simulink model "InverseDynamicsController"  (R2020b)
settings: Solver=FixedStepAuto  StartTime=0.0  StopTime=42  RelTol=1e-3
settings Model: Creator=Riley  LastModifiedBy=Riley

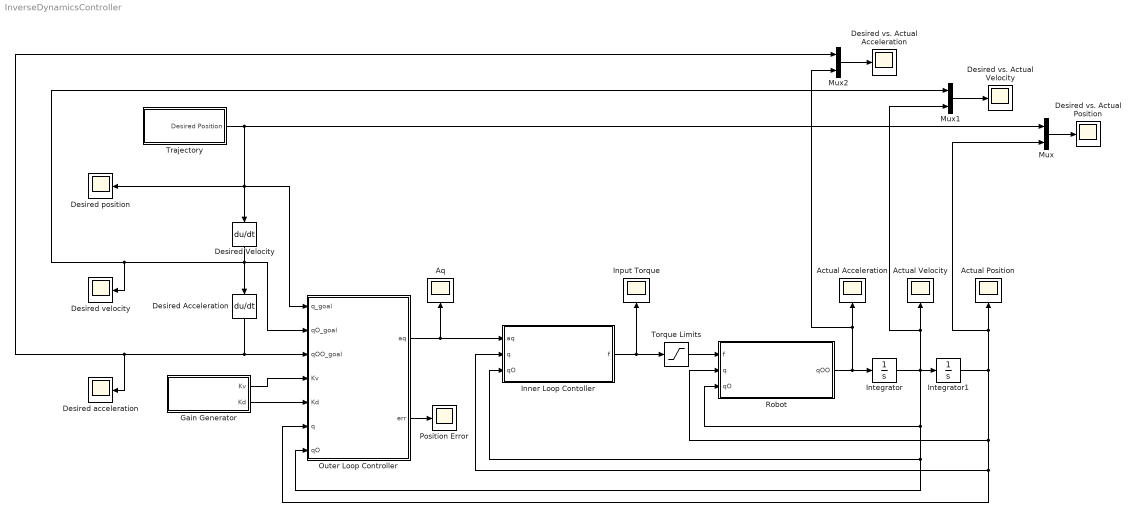
== system InverseDynamicsController ==
  Actual Acceleration : Scope
  Actual Position : Scope
  Actual Velocity : Scope
  Aq : Scope
  Desired Acceleration : Derivative
  Desired Velocity : Derivative
  Desired acceleration : Scope
  Desired position : Scope
  Desired velocity : Scope
  Desired vs. Actual Acceleration : Scope
  Desired vs. Actual Position : Scope
  Desired vs. Actual Velocity : Scope
  Gain Generator : Subsystem
  Inner Loop Contoller : MATLAB Function  TreatAsAtomicUnit=on
  Input Torque : Scope
  Integrator : Integrator  InitialCondition=[0,0,0]
  Integrator1 : Integrator  InitialCondition=[0,0,0]
  Mux : Mux  Inputs=2
  Mux1 : Mux  Inputs=2
  Mux2 : Mux  Inputs=2
  Outer Loop Controller : MATLAB Function  TreatAsAtomicUnit=on
  Position Error : Scope
  Robot : MATLAB Function  TreatAsAtomicUnit=on
  Torque Limits : Saturate  UpperLimit=4000000  LowerLimit=-4000000
  Trajectory : Subsystem
  wires:
  Gain Generator/2(Kd) -> Outer Loop Controller/5(Kd)
  Gain Generator/1(Kv) -> Outer Loop Controller/4(Kv)
  Trajectory/1(Desired Position) -> Mux/1, Desired position/1, Outer Loop Controller/1(q_goal), Desired Velocity/1
  Desired Acceleration/1 -> Desired acceleration/1, Mux2/1, Outer Loop Controller/3(qOO_goal)
  Desired Velocity/1 -> Mux1/1, Desired velocity/1, Outer Loop Controller/2(qO_goal), Desired Acceleration/1
  Outer Loop Controller/2(err) -> Position Error/1
  Outer Loop Controller/1(aq) -> Aq/1, Inner Loop Contoller/1(aq)
  Inner Loop Contoller/1(f) -> Torque Limits/1, Input Torque/1
  Robot/1(qOO) -> Actual Acceleration/1, Mux2/2, Integrator/1
  Integrator1/1 -> Robot/2(q), Inner Loop Contoller/2(q), Outer Loop Controller/6(q), Mux/2, Actual Position/1
  Mux/1 -> Desired vs. Actual Position/1
  Torque Limits/1 -> Robot/1(f)
  Mux1/1 -> Desired vs. Actual Velocity/1
  Integrator/1 -> Inner Loop Contoller/3(qO), Outer Loop Controller/7(qO), Robot/3(qO), Mux1/2, Actual Velocity/1, Integrator1/1
  Mux2/1 -> Desired vs. Actual Acceleration/1

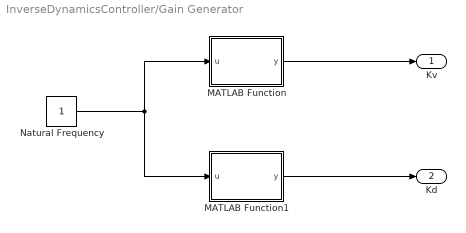
== system InverseDynamicsController/Gain Generator ==
  MATLAB Function : MATLAB Function  TreatAsAtomicUnit=on
  MATLAB Function1 : MATLAB Function  TreatAsAtomicUnit=on
  Natural Frequency : Constant
  Kv : Outport
  Kd : Outport  Port=2
  wires:
  Natural Frequency/1 -> MATLAB Function1/1(u), MATLAB Function/1(u)
  MATLAB Function/1(y) -> Kv/1
  MATLAB Function1/1(y) -> Kd/1

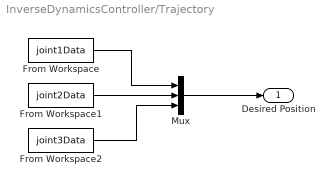
== system InverseDynamicsController/Trajectory ==
  From Workspace : FromWorkspace  VariableName=joint1Data
  From Workspace1 : FromWorkspace  VariableName=joint2Data
  From Workspace2 : FromWorkspace  VariableName=joint3Data
  Mux : Mux  Inputs=3
  Desired Position : Outport
  wires:
  From Workspace2/1 -> Mux/3
  From Workspace1/1 -> Mux/2
  From Workspace/1 -> Mux/1
  Mux/1 -> Desired Position/1

== matlab function InverseDynamicsController/Gain Generator/MATLAB Function1 ==
  data: u input; y output
function y = K0matrix(u)
%K0matrix calculates the K0 gain matrix given the user specified natural
%frequency

%y = K0matrix(u) where u is the inputted user-specified natural frequency
%scalar and y is the outputted K0 gain matrix

    y = [u*u, 0, 0;
         0, u*u, 0;
         0, 0, u*u];
    
end

== matlab function InverseDynamicsController/Gain Generator/MATLAB Function ==
  data: u input; y output
function y = K1matrix(u)
%K1matrix calculates the K1 gain matrix given the user specified natural
%frequency

%y = K1matrix(u) where u is the inputted user-specified natural frequency
%scalar and y is the outputted K1 gain matrix

    y = [2*u, 0, 0;
         0, 2*u, 0;
         0, 0, 2*u];
    
end

== matlab function InverseDynamicsController/Outer Loop Controller ==
  data: q_goal input; aq output; qO_goal input; qOO_goal input; Kv input; Kd input; q input; qO input; err output
function [aq, err] = outerLoopController(q_goal, qO_goal, qOO_goal, Kv, Kd, q, qO)
%outerLoopController calculates inverse dynamics controller aq component

%[aq, err] = outerLoopController(q_goal, qO_goal, qOO_goal, q, qO, Kv, Kd)
%where q_goal, qO_goal, and qOO_goal are input 3x1 column vectors of the
%respective desired position, velocity, and acceleration of the manipulator
%joints in the form [joint 1, joint 2, joint 3]', Kv and Kd are input 3x3
%matrices of the respective gains in the form:     [K, 0, 0;
%                                                   0, K, 0
%                                                   0, 0, K]
%q and qO are input 3x1 column vectors of the respective actual position
%and velocity of the manipulator joints in the form [joint 1, joint 2,
%joint 3]', aq is an output 3x1 column vector of the acceleration input to
%the inner control loop, and err is an output 3x1 column vector of the 
%current difference between the desired and actual joint positions

    %computing aq
    aq = qOO_goal-(Kd*(q-q_goal))-(Kv*(qO-qO_goal));
    
    %computing error
    err = q_goal - q;

end

== matlab function InverseDynamicsController/Inner Loop Contoller ==
  data: aq input; q input; qO input; f output
function f = innerLoopController(aq, q, qO)
%innerLoopController calculates reRACKer inverse dynamics

%f = innerLoopController(aq, q, qO) where aq is an input 3x1 column vector
%of the outer-loop controller output, q and qO are input 3x1 column vectors
%of the respective actual joint position and velocity of the manipulator,
%and f is an output 3x1 column vector of the resulting torque commanded to
%the manipulator. All vectors are of the form [joint 1, joint 2, joint 3]'.

    %calculating joint torque
    f = dynamicForces(q, qO, aq);

end

== matlab function InverseDynamicsController/Robot ==
  data: f input; q input; qO input; qOO output
function qOO = forwardDynamics(f, q, qO)
%forwardDynamics calculates reRACKer forward dynamics

%qOO = forwardDynamics(f, q, qO) where f is an input 3x1 column vector of
%the torque commanded to the manipulator, q and qO are input 3x1 column
%vectors of the respective actual joint position and velocity of the
%manipulator, and qOO is an output 3x1 column vector of the actual joint
%acceleration of the manipulator. All vectors are of the form [joint 1,
%joint 2, joint 3]'.


    %----------------------------------------------------------------------
    %extracting input vectors for readability
    %----------------------------------------------------------------------
    
    %extracting joint torques
    Tt1 = f(1);                                                             %revolute joint 1 torque
    Tt2 = f(2);                                                             %prismatic joint 2 torque
    Tt3 = f(3);                                                             %prismatic joint 3 torque
    
    %extracting joint positions
    T1 = q(1);                                                              %revolute joint 1 angle
    D2 = q(2);                                                              %prismatic joint 2 distance
    D3 = q(3);                                                              %prismatic joint 3 distance
    
    %extracting joint velocities
    T1_O = qO(1);                                                           %revolute joint 1 velocity
    D2_O = qO(2);                                                           %prismatic joint 2 velocity
    D3_O = qO(3);                                                           %prismatic joint 3 velocity
    
    
    %----------------------------------------------------------------------
    %defining manipulator physical parameters
    %----------------------------------------------------------------------

    %defining physical manipulator link lengths of SolidWorks Model
    L1 = 55;                                                                %length of link 1 in inches
    L2 = 65;                                                                %length of link 2 in inches
    L3 = 32;                                                                %length of link 3 in inches

    %defining physical manipulator link masses of SolidWorks Model
    m1 = 69.05;                                                             %mass of link 1 in pounds
    m2 = 51.33;                                                             %mass of link 2 in pounds
    m3 = 18.73;                                                             %mass of link 3 in pounds

    %defining physical manipulator link CoMs of SolidWorks Model
    swCoM1 = [0,  24.86, 0];                                                %SolidWorks link 1 CoM WRT part [x, y, z] frame
    swCoM2 = [33.51, 0, 0];                                                 %SolidWorks link 2 CoM WRT part [x, y, z] frame
    swCoM3 = [0, 16, 0];                                                    %SolidWorks link 3 CoM WRT part [x, y, z] frame

    %defining physical manipulator link inertias of SolidWorks Model
    swI1 = [24407.21, 1976.07, 23918.19];                                   %SolidWorks link 1 inertia WRT assembly [x, y, z] frame
    swI2 = [848.56,  21959.25, 21658.21];                                   %SolidWorks link 2 inertia WRT assembly [x, y, z] frame
    swI3 = [2028.91, 164.39, 1976.88];                                      %SolidWorks link 3 inertia WRT assembly [x, y, z] frame

    %defining physical manipulator link inertia matrices (converted from SolidWorks frames to DH frames)
    I1 = [swI1(3), 0, 0; 0, swI1(2), 0; 0, 0, swI1(1)];                     %inertia matrix of link 1 WRT DH frame 1 (with frame 1 translated to link 1 CoM) 
    I2 = [swI2(3), 0, 0; 0, swI2(1), 0; 0, 0, swI2(2)];                     %inertia matrix of link 2 WRT DH frame 2 (with frame 2 translated to link 2 CoM)
    I3 = [swI3(3), 0, 0; 0, swI3(1), 0; 0, 0, swI3(2)];                     %inertia matrix of link 3 WRT DH frame 3 (with frame 3 translated to link 3 CoM)

    %defining gravity in IPS units
    g = 386.09;
    
    
    %----------------------------------------------------------------------
    %constructing terms used in equations
    %----------------------------------------------------------------------

    %constructing inertia values
    I1yy = I1(2, 2);
    I2zz = I2(3, 3);
    I3zz = I3(3, 3);

    %constructing length scalars to link i CoM WRT joint i+1
    Lc1 = L1 - swCoM1(2);                                                   %length from joint 2 to link 1 CoM
    Lc2 = L2 - swCoM2(1);                                                   %length from joint 3 to link 2 CoM
    Lc3 = L3 - swCoM3(2);                                                   %length from end effector to link 3 CoM

    
    %----------------------------------------------------------------------
    %calculating joint accelerations using dynamic equations
    %----------------------------------------------------------------------
    
    %calculating qOO = (T - C(q,qO)qO - g)/D(q)
    D3_OO = (Tt3 - (m3*g))/m3;
    D2_OO = (Tt2 - (((Lc2*m2)-(L1*m2)-(L1*m3))*(T1_O*T1_O)))/(m2+m3);
    T1_OO = (Tt1 - (((L1*m2)+(L1*m3)-(Lc1*m2)-(Lc1*m3)+(Lc2*m3))...
        *(2*D2_O*T1_O)))/((L1*L1*m1)+(L1*L1*m2)+(L1*L1*m3)+(Lc1*Lc1*m1)...
        -(2*L1*Lc1*m1)-(L1*Lc1*m2)-(L1*Lc1*m3)-(L1*Lc2*m2)+(L1*Lc2*m3)...
        +(Lc1*Lc2*m2)+I1yy+I2zz+I3zz);

    %formatting return
    qOO = [double(T1_OO), double(D2_OO), double(D3_OO)]';
end
